simulink model "FULLsystem"  (R2024b)
settings: Solver=FixedStepAuto  StartTime=0.0  StopTime=inf  RelTol=1e-3
InitFcn:
  | close all
  | QAM_ORDER = 64;
undefined symbols (not defined in the file or in its folder): QAM
libraries: commrfcorlib x3, commsync2 x2, commrflib2 x2, commfilt2 x2, commdigbbndam3 x2, commchan3 x1
settings Model: Creator=J_mas  LastModifiedBy=J_mas

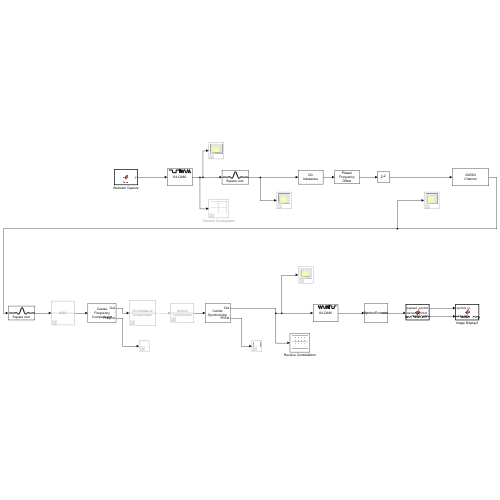
[thumbnail: Simulink's stored preview of the top-level diagram]
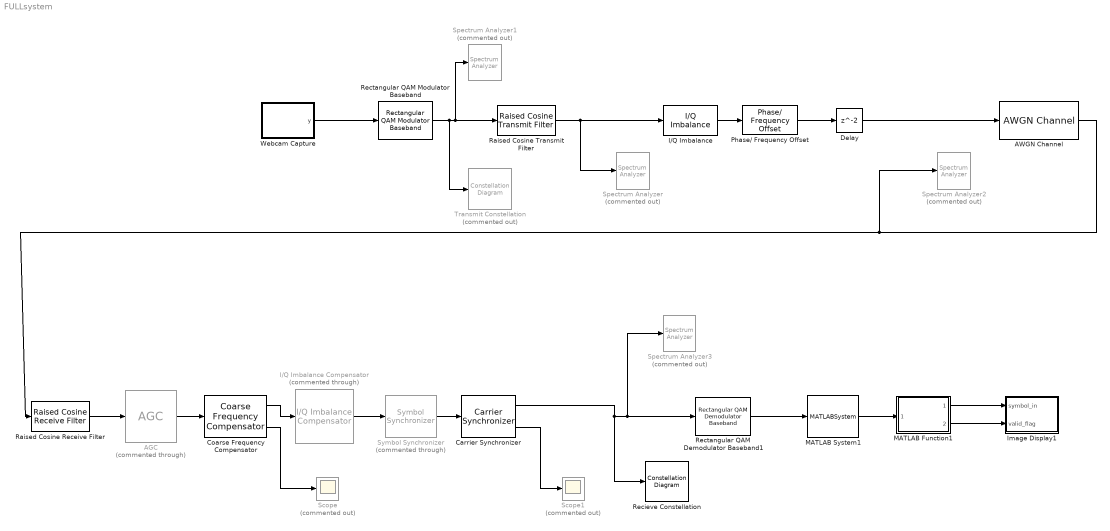
== system FULLsystem ==
  AGC : commrfcorlib/AGC  Commented=through  LegacyMode=off  DetectorMethod=Rectifier  LoopMethod=Linear  UpdatePeriod=100  StepSize=0.1  AdaptationStepSize=0.01  DesiredOutputPower=1  AveragingLength=100  MaximumGain=30  MaxPowerGain=60  GainOutputPort=off  InputPowerOutputPort=off  SimulateUsing=Interpreted execution
  AWGN Channel : commchan3/AWGN Channel  LegacyMode=off  NoiseMethod="Signal to noise ratio  (SNR)"  noiseMode="Signal to noise ratio  (SNR)"  EbNo=10  EsNo=10  SNR=30  BitsPerSymbol=1  SignalPower=1  SamplesPerSymbol=1  SymbolPeriod=1  VarianceSource=Parameter  Variance=1  RandomStream=Global stream  Seed=67  SimulateUsing=Code generation
  Carrier Synchronizer : commsync2/Carrier Synchronizer  Modulation=QAM  ModulationPhaseOffset=Auto  CustomPhaseOffset=0  SamplesPerSymbol=8  DampingFactor=1  NormalizedLoopBandwidth=0.0005  EstimatedPhaseErrorOutputPort=on  SimulateUsing=Code generation
  Coarse Frequency Compensator : commrfcorlib/Coarse Frequency Compensator  Modulation=QAM  Algorithm=FFT-based  FrequencyResolution=10  MaximumFrequencyOffset=5e3  SamplesPerSymbol=4  EstimatedFreqOffsetPort=on  SimulateUsing=Code generation
      settings: LibrarySourceBlock=|
      | commsync2/Coarse Frequency
      | Compensator
  Delay : Delay  InitialCondition=0
  I/Q Imbalance : commrflib2/I//Q Imbalance  ampImbal=2  phsImbal=5  Idc=0  Qdc=0
  I/Q Imbalance Compensator : commrfcorlib/I//Q Imbalance Compensator  Commented=through  CoefficientSource=Estimated from input signal  InitialCoefficient=0 + 0j  StepSizeSource=Property  StepSize=0.0000001  AdaptInputPort=off  CoefficientOutputPort=off  SimulateUsing=Code generation
  Image Display1 : MATLAB Function  TreatAsAtomicUnit=on
  MATLAB Function1 : MATLAB Function  TreatAsAtomicUnit=on
  MATLAB System1 : MATLABSystem  System=SymbolExtractor  SimulateUsing=Code generation
      mask Type: SymbolExtractor
      mask Display:
      | disp('SymbolExtractor');
      | port_label('input',1,'in');
      | port_label('output',1,'out');
  Phase/ Frequency Offset : commrflib2/Phase// Frequency Offset  phaseOffset=40  freqPort=off  freqOffset=200
  Raised Cosine Receive Filter : commfilt2/Raised Cosine Receive Filter  filtType=Square root  R=0.2  filtSpan=10  N=8  downFactor=8  downOffset=0  filterGain=1  InputProcessing=Columns as channels (frame based)  RateOptions=Enforce single-rate processing  framing=Mute  checkCoeff=off  variableName=rcRxFilt  currentFiltSpan=10  D=5  inputOffset=0  sampMode=Mute  saveAsFlag=0  rateMode=Downsampling  checkGain=Normalized  launchFVT=on  roundingMode=Floor  overflowMode=off  coeffDataTypeStr=Inherit: Same word length as input  coeffMin=[]  coeffMax=[]  coeffLastDataTypeStr=Inherit: Same word length as input  accumDataTypeStr=Inherit: Same as product output  accumLastDataTypeStr=Inherit: Same as product output  outputDataTypeStr=Inherit: Same as accumulator  outputMin=[]  outputMax=[]  outputLastDataTypeStr=Inherit: Same as accumulator
  Raised Cosine Transmit Filter : commfilt2/Raised Cosine Transmit Filter  filtType=Square root  R=0.2  filtSpan=10  N=8  filterGain=1  InputProcessing=Columns as channels (frame based)  RateOptions=Enforce single-rate processing  framing=Mute  checkCoeff=off  variableName=rcTxFilt  checkGain=Normalized  sampMode=Mute  saveAsFlag=0  currentFiltSpan=10  D=(10)/2  launchFVT=on  roundingMode=Floor  overflowMode=off  coeffDataTypeStr=Inherit: Same word length as input  coeffMin=[]  coeffMax=[]  coeffLastDataTypeStr=Inherit: Same word length as input  outputDataTypeStr=Inherit: Same as accumulator  outputMin=[]  outputMax=[]  outputLastDataTypeStr=Inherit: Same as accumulator
  Recieve Constellation : ConstellationDiagram  WindowPosition=[1152.000000,229.000000,367.000000,296.000000,]  Visible=on  ScopeFrameLocation=window  SamplesPerSymbol=8  SymbolsToDisplaySource=Property  SymbolsToDisplay=100  ReferenceConstellation=64-QAM  XLimits=[-3.19,3.19]  YLimits=[-2.54,2.54]
  Rectangular QAM Demodulator Baseband1 : commdigbbndam3/Rectangular QAM Demodulator Baseband  M=QAM_ORDER  OutType=Integer  DecType=Hard decision  VarSource=Dialog  Variance=1  Dec=Gray  Mapping=[0:15]  PowType=Min. distance between symbols  MinDist=2  AvgPow=1  PeakPow=1  Ph=0  outDtype1=Inherit via internal rule  outDtype2=uint8  derotateFactorWordLen=16  derotateFactorDataTypeStr=Inherit: Same word length as input  derotateFactorLastDataTypeStr=Inherit: Same word length as input  denormFactorWordLen=16  denormFactorDataTypeStr=Inherit: Same word length as input  denormFactorLastDataTypeStr=Inherit: Same word length as input  prodOutWordLen=32  prodOutOverflowMode=Wrap  prodOutRoundingMode=Floor  prodOutOvFlMode=off  prodOutOvFlModeLastStrValue=off  sumWordLen=32
  Rectangular QAM Modulator Baseband : commdigbbndam3/Rectangular QAM Modulator Baseband  M=QAM_ORDER  InType=Integer  Enc=Gray  Mapping=[0:15]  PowType=Min. distance between symbols  MinDist=2  AvgPow=1  PeakPow=1  Ph=0  outDtype=double  outWordLen=16  outUDDataType=sfix(16)  outFracLenMode=Best precision  outFracLen=15  outDataTypeStr=double  outLastDataTypeStr=double
  Scope : Scope  Commented=on
  Scope1 : Scope  Commented=on
  Spectrum Analyzer : SpectrumAnalyzer  Commented=on  WindowPosition=[766.000000,145.000000,800.000000,500.000000,]  Visible=on  ScopeFrameLocation=window  WindowInvariantSamplesPerUpdate=on  Span=320000  StartFrequency=-160000  StopFrequency=160000
  Spectrum Analyzer1 : SpectrumAnalyzer  Commented=on  WindowPosition=[76.000000,141.000000,800.000000,500.000000,]  Visible=on  ScopeFrameLocation=window  WindowInvariantSamplesPerUpdate=on  Span=40000  StartFrequency=-20000  StopFrequency=20000  YLimits=[2.7638,43.4449]
  Spectrum Analyzer2 : SpectrumAnalyzer  Commented=on  WindowPosition=[132.000000,174.000000,800.000000,500.000000,]  Visible=on  ScopeFrameLocation=window  WindowInvariantSamplesPerUpdate=on  Span=320000  StartFrequency=-160000  StopFrequency=160000  YLimits=[-40.80971034,36.15019353]
  Spectrum Analyzer3 : SpectrumAnalyzer  Commented=on  WindowPosition=[634.000000,148.000000,800.000000,500.000000,]  Visible=on  ScopeFrameLocation=window  WindowInvariantSamplesPerUpdate=on  YLimits=[0.325,45.0986]
  Symbol Synchronizer : commsync2/Symbol Synchronizer  Commented=through  Modulation=PAM/PSK/QAM  TimingErrorDetector=Gardner (non-data-aided)  SamplesPerSymbol=2  DampingFactor=1  NormalizedLoopBandwidth=0.02  DetectorGain=2.7  TimingErrorOutputPort=off  SimulateUsing=Code generation
  Transmit Constellation : ConstellationDiagram  Commented=on  WindowPosition=[145.000000,119.000000,313.000000,159.000000,]  Visible=on  ScopeFrameLocation=window  SamplesPerSymbol=8  SymbolsToDisplaySource=Property  SymbolsToDisplay=100  ReferenceConstellation=64-QAM  XLimits=[-3.19,3.19]  YLimits=[-2.54,2.54]
  Webcam Capture : MATLAB Function  TreatAsAtomicUnit=on  SystemSampleTime=1/40000
  wires:
  Rectangular QAM Modulator Baseband/1 -> Transmit Constellation/1, Spectrum Analyzer1/1, Raised Cosine Transmit Filter/1
  Raised Cosine Transmit Filter/1 -> Spectrum Analyzer/1, I/Q Imbalance/1
  I/Q Imbalance/1 -> Phase/ Frequency Offset/1
  Symbol Synchronizer/1 -> Carrier Synchronizer/1
  Coarse Frequency Compensator/1 -> I/Q Imbalance Compensator/1
  MATLAB Function1/1(payload_symbol) -> Image Display1/1(symbol_in)
  MATLAB Function1/2(frame_valid) -> Image Display1/2(valid_flag)
  Phase/ Frequency Offset/1 -> Delay/1
  AWGN Channel/1 -> Spectrum Analyzer2/1, Raised Cosine Receive Filter/1
  MATLAB System1/1 -> MATLAB Function1/1(demod_symbol)
  AGC/1 -> Coarse Frequency Compensator/1
  Raised Cosine Receive Filter/1 -> AGC/1
  I/Q Imbalance Compensator/1 -> Symbol Synchronizer/1
  Coarse Frequency Compensator/2 -> Scope/1
  Carrier Synchronizer/2 -> Scope1/1
  Delay/1 -> AWGN Channel/1
  Carrier Synchronizer/1 -> Recieve Constellation/1, Spectrum Analyzer3/1, Rectangular QAM Demodulator Baseband1/1
  Webcam Capture/1(y) -> Rectangular QAM Modulator Baseband/1
  Rectangular QAM Demodulator Baseband1/1 -> MATLAB System1/1

== matlab function FULLsystem/Image Display1 ==
  data: symbol_in input; valid_flag input
function reconstruct_image(symbol_in, valid_flag) %#codegen
    coder.extrinsic('imshow', 'figure', 'drawnow', 'title');
    
    persistent imgBuffer symbolCount fig initialized IMG_ROWS IMG_COLS FRAME_LEN
    
    if isempty(initialized)
        % Define image size here OR pass as parameters if needed
        IMG_ROWS = 100;
        IMG_COLS = 100;
        
        FRAME_LEN = IMG_ROWS * IMG_COLS;
        
        imgBuffer = uint8(zeros(IMG_ROWS, IMG_COLS));
        symbolCount = 0;
        
        fig = figure('Name', 'Received Image');
        initialized = true;
    end
    
    % Only accumulate if we have valid payload data
    if valid_flag
        symbolCount = symbolCount + 1;
        
        if symbolCount <= FRAME_LEN
            imgBuffer(symbolCount) = uint8(symbol_in * 4);
        end
        
        % Display complete frame
        if symbolCount == FRAME_LEN
            %imshow(imgBuffer);
            imshow(imresize(imgBuffer, 4), []);  % 4x bigger display, no interpolation needed for uint8
            title('Received Image');
            drawnow;
            
            % Reset for next frame
            symbolCount = 0;
        end
    end
end

== matlab function FULLsystem/MATLAB Function1 ==
  data: demod_symbol input size=1; payload_symbol output uint8 size=1; frame_valid output boolean size=1

function [payload_symbol, frame_valid] = barkerFrameDetector(demod_symbol)
%#codegen

% ===== Image dimensions =====
IMG_ROWS = uint32(100);
IMG_COLS = uint32(100);
PAYLOAD_LIMIT = IMG_ROWS * IMG_COLS;
% ============================

% Force fixed scalar input
sym_in = uint8(demod_symbol(1,1));

% Explicit scalar outputs
payload_symbol = uint8(0);
frame_valid    = logical(false);

persistent preambleBuffer collecting payloadCounter
if isempty(collecting)
    preambleBuffer = zeros(13,1,'uint8');
    collecting     = false;
    payloadCounter = uint32(0);
end

PREAMBLE = uint8([63;63;63;63;63;0;0;63;63;0;63;0;63]);

if ~collecting

    % Shift buffer
    for i = 1:12
        preambleBuffer(i) = preambleBuffer(i+1);
    end
    preambleBuffer(13) = sym_in;

    % Compare with preamble
    matches = uint8(0);
    for i = 1:13
        if preambleBuffer(i) == PREAMBLE(i)
            matches = matches + uint8(1);
        end
    end

    % Start collecting if matched
    if matches >= 11
        collecting     = true;
        payloadCounter = uint32(0);
    end

else

    payloadCounter = payloadCounter + 1;

    if payloadCounter <= PAYLOAD_LIMIT
        payload_symbol = sym_in;
        frame_valid    = true;
    end

    if payloadCounter >= PAYLOAD_LIMIT
        collecting     = false;
        payloadCounter = uint32(0);
    end
end

end

== matlab function FULLsystem/Webcam Capture ==
  data: y output
function y = fcn() %#codegen
    coder.extrinsic('webcam', 'snapshot', 'imresize', 'rgb2gray', 'imshow', 'tic', 'toc', 'fprintf');

    persistent cam packetBuffer packetIndex initialized startTime symbolCount

    y = uint8(0); % Output type should match Modulator input (usually integer)

    % Barker code parameters
    BARKER_LENGTH = 13; % Length-13 Barker code for good autocorrelation
    IMG_ROWS = 100;
    IMG_COLS = 100;
    PAYLOAD_LENGTH = IMG_ROWS * IMG_COLS;

    PACKET_LENGTH = BARKER_LENGTH + PAYLOAD_LENGTH;

    if isempty(initialized)
        cam = webcam(1);
        startTime = tic;

        % Buffer now holds complete packets (preamble + payload)
        packetBuffer = uint8(zeros(PACKET_LENGTH, 1));
        packetIndex = PACKET_LENGTH + 1; % Start beyond buffer to trigger capture
        symbolCount = 0;
        initialized = true;
    end

    % When we've transmitted the entire packet, capture a new frame
    if packetIndex > PACKET_LENGTH
        % Capture and process webcam image
        rawImg = snapshot(cam);
        imgResized = imresize(rawImg, [IMG_ROWS, IMG_COLS]);
        imgGrayRaw = rgb2gray(imgResized);
        %imshow(imgGrayRaw);
        %title('Transmitted Image');
        %drawnow;


        imgGray = uint8(zeros(IMG_ROWS, IMG_COLS));
        imgGray = imgGrayRaw;

        % Flatten the image and convert to 6-bit symbols (0-63)
        temp = reshape(imgGray, PAYLOAD_LENGTH, 1);
        payload = uint8(floor(double(temp) / 4)); % Map 0-255 to 0-63

        % Create Barker code preamble
        % Standard 13-bit Barker: [1 1 1 1 1 -1 -1 1 1 -1 1 -1 1]
        % Map to 6-bit symbols: use 63 for '1' and 0 for '-1' for good separation
        barker_preamble = uint8([63 63 63 63 63 0 0 63 63 0 63 0 63]');

        % Construct packet: [Preamble | Payload]
        packetBuffer(1:BARKER_LENGTH) = barker_preamble;
        packetBuffer(BARKER_LENGTH+1:PACKET_LENGTH) = payload;

        % Reset index to start of packet
        packetIndex = 1;

        % Statistics
        elapsedTime = toc(startTime);
        symbolRate = symbolCount / elapsedTime;
        fprintf('Symbol Rate: %.2f symbols/sec\n', symbolRate);
        fprintf('Packet Rate: %.2f frames/sec\n', symbolCount / (PACKET_LENGTH * elapsedTime));
    end

    % Output one symbol per call
    if packetIndex <= PACKET_LENGTH
        y = packetBuffer(packetIndex);
        packetIndex = packetIndex + 1;
        symbolCount = symbolCount + 1;
    end
end
